simulink model "CRH2forBenchmark"  (R2014a)
settings: Solver=ode3  StartTime=0.0  StopTime=1  FixedStep=1e-5  RelTol=1e-3
PostLoadFcn:
  | , if any(exist('dsrtsu_mdlpostloadfcn', 'file') == [2, 3, 6]), try dsrtsu_mdlpostloadfcn('Execute', bdroot); catch fprintf('Error in PostLoadFcn (dsrtsu_mdlpostloadfcn) for model "%s":\n %s\n', bdroot, lasterr); end, end,
values from neighbouring files (symbols this model uses):
  Cd = 0.016    [CRH2forBenchmark.mat]
  Lm = 0.032848    [CRH2forBenchmark.mat]
  Ln = 0.002    [CRH2forBenchmark.mat]
  Lr = 0.034142    [CRH2forBenchmark.mat]
  Ls = 0.0342654    [CRH2forBenchmark.mat]
  np = 2    [CRH2forBenchmark.mat]
  Rd = 6000    [CRH2forBenchmark.mat]
  Rn = 0.2    [CRH2forBenchmark.mat]
  Rr = 0.146    [CRH2forBenchmark.mat]
  Rs = 0.144    [CRH2forBenchmark.mat]
  ts = 1e-05    [CRH2forBenchmark.mat]
undefined symbols (not defined in the file): J, KIM, KIT, KPM, KPT, phir, Ts, Vge
libraries: simulink x10
(part 1 of 3)
settings Model: DSRTSU_INTERNAL_RTI_VER=450  DSRTSU_INTERNAL_RTI_TYPE=rti1007  DSRTSU_INTERNAL_RTIFPGA=40  BufferReuse=off  Creator=超  LastModifiedBy=卍
settings SolverCC: AlgebraicLoopSolver=LineSearch
settings DataIOCC: SignalLoggingSaveFormat=ModelDataLogs
settings OptimizationCC: BlockReduction=off  OptimizeBlockIOStorage=off  BufferReuse=off  GlobalBufferReuse=off  ExpressionFolding=off  LocalBlockOutputs=off
settings DebuggingCC: MultiTaskDSMMsg=warning  MultiTaskCondExecSysMsg=none
settings HardwareCC: ProdIntDivRoundTo=Zero  ProdEndianess=BigEndian  ProdHWDeviceType=Generic->Custom  TargetIntDivRoundTo=Zero  TargetEndianess=BigEndian  TargetHWDeviceType=Generic->Custom
settings RTWCC: SystemTargetFile=rti1007.tlc  MakeCommand=make_rti  TemplateMakefile=rti1007.tmf  Description=dSPACE DS1007 Hardware Platform  ProcessScript=rti1007_make_rtw_hook  IncludeERTFirstTime=on
settings STFCustomTargetCC: ParMdlRefBuildCompliant=on  ConcurrentExecutionCompliant=off  MatFileLogging=on  SystemTargetFile=rti1007.tlc
settings GRTTargetCC: CompOptLevelCompliant=off  ConcurrentExecutionCompliant=off  CombineOutputUpdateFcns=off  CPPClassGenCompliant=off  GRTInterface=on  ExtModeMexFile=noextcomm

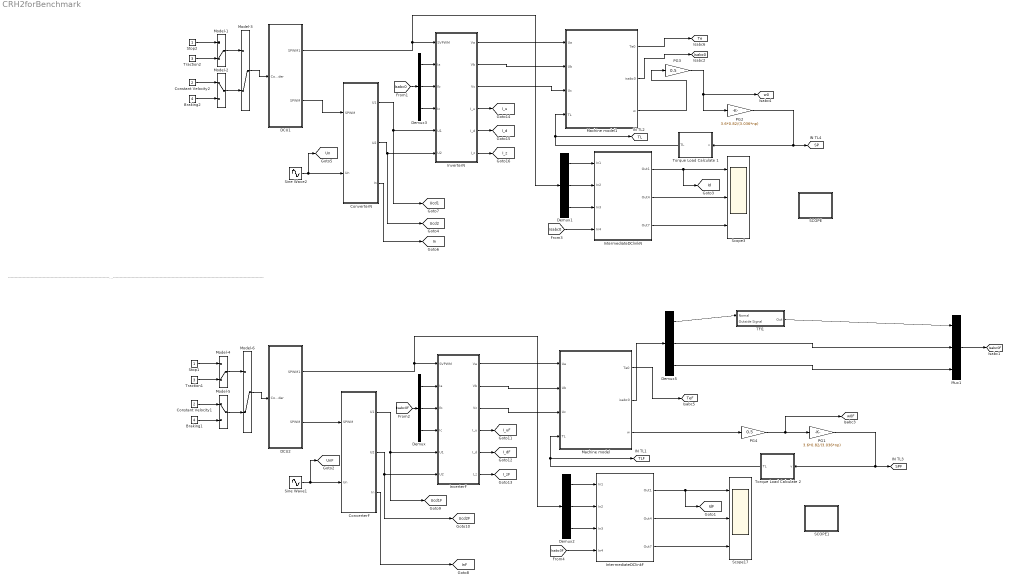
== system CRH2forBenchmark ==
  note: ------------------------------------------------------------------------------------------------------------------------------------------------------------------------------------------------------------------------------------------------------------------------------------------------------------------------------------------------------------------------------------------------------------------------------------------------------------------------------------------------------------------------------------------------------------------------------------------------------------------------------------------------------------------------------------------------------------------------------------------------------------------------------------------------------------------------------------------------------------------
  " Constant Velocity1" : Constant  Value=2
  " Constant Velocity2" : Constant  Value=2
  Braking1 : Constant  Value=4
  Braking2 : Constant  Value=4
  ConverterF : Subsystem
  ConverterN : Subsystem
  DCU1 : Subsystem  mask{sfcnParam1=KIM, sfcnParam2=KIT, sfcnParam3=KPM, sfcnParam4=KPT, sfcnParam5=Ts, sfcnParam6=Vge, sfcnParam7=np, sfcnParam8=phir}
      mask prompts: sfcnParam1 "KIM:"; sfcnParam2 "KIT:"; sfcnParam3 "KPM:"; sfcnParam4 "KPT:"; sfcnParam5 "Ts:"; sfcnParam6 "Vge:"; sfcnParam7 "np:"; sfcnParam8 "phir:"
      mask help: Simulink:masks:GenSFuncDesc_MD
      mask Help: eval('feval(''rtwprivate'',''rtwhelpview'',''rtw_sfcn_block'')');
      mask Display: fprintf('Traction Control\nUnit(TCU)')
  DCU2 : Subsystem  mask{sfcnParam1=KIM, sfcnParam2=KIT, sfcnParam3=KPM, sfcnParam4=KPT, sfcnParam5=Ts, sfcnParam6=Vge, sfcnParam7=np, sfcnParam8=phir}
      mask prompts: sfcnParam1 "KIM:"; sfcnParam2 "KIT:"; sfcnParam3 "KPM:"; sfcnParam4 "KPT:"; sfcnParam5 "Ts:"; sfcnParam6 "Vge:"; sfcnParam7 "np:"; sfcnParam8 "phir:"
      mask help: Simulink:masks:GenSFuncDesc_MD
      mask Help: eval('feval(''rtwprivate'',''rtwhelpview'',''rtw_sfcn_block'')');
      mask Display: fprintf('Traction Control\nUnit(TCU)')
  Demux{,1..3,5} (5 alike) : Demux  Outputs=3
  IntermediateDClinkF : Subsystem
      mask help: Simulink:masks:GenSFuncDesc_MD
      mask Help: eval('feval(''rtwprivate'',''rtwhelpview'',''rtw_sfcn_block'')');
  IntermediateDClinkN : Subsystem
      mask help: Simulink:masks:GenSFuncDesc_MD
      mask Help: eval('feval(''rtwprivate'',''rtwhelpview'',''rtw_sfcn_block'')');
  InverterF : Subsystem
  InverterN : Subsystem
  Machine model : Subsystem
  Machine model1 : Subsystem
  Model-{1,3..4,6} (4 alike) : ManualSwitch  CurrentSetting=0
  Model-2 : ManualSwitch
  Model-5 : ManualSwitch
  Mux1 : Mux  Inputs=3
  PG1 : Gain  Gain=3.6*0.82/(3.036*np)
  PG2 : Gain  Gain=3.6*0.82/(3.036*np)
  PG3 : Gain  Gain=0.5
  PG4 : Gain  Gain=0.5
  SCOPE : Subsystem
  SCOPE1 : Subsystem
  Scope17 : Scope  NumInputPorts=3
      settings: TickLabels=on  TimeRange=5  YMin=0~-110~-130  YMax=130~110~0  SaveName=AF  SampleInput=on  SampleTime=ts
  Scope3 : Scope  NumInputPorts=3
      settings: TickLabels=on  TimeRange=5  YMin=0~-110~-130  YMax=130~110~0  SaveName=A  SampleInput=on  SampleTime=ts
  Sine Wave1 : Sin  Amplitude=2121  Frequency=50*pi*2  SampleTime=ts
  Sine Wave2 : Sin  Amplitude=2121  Frequency=50*pi*2  SampleTime=ts
  Stop1 : Constant
  Stop2 : Constant
  TFI1 : Subsystem  mask(TFI){FaultType=SET anolog mode fault, FaultInjectionTime=1, Apq=[25 -500 -1000], TH=3.5, InvertBit=1, Register_Ts=1e-5, NoiseSelec=on, NoiseFault=[0.001 1e-5 23341], Comp_ConV=[23341], AddMux=Add}
      mask prompts: FaultType "Fault Type"; FaultInjectionTime "Fault Injection Time"; Apq "A,p,q"; InvertBit "Invert Bit"; NoiseSelec "Noise Disturbance"; NoiseFault "Noise Disturbance(Noise power,Sample time,Seed)"; Comp_ConV "Compare Constant Value"; AddMux "Add or Mux(outside signal)"
      mask help:
      | TCU Fault Injector (TFI)
      | 1.Fault Injection Time:Set the parameter of Fault-Inject Time;
      | 2.A,p,q:(Amplitude parameter, time parameter, time parameter)Setting analog model fault injection(Double exponential model ) signal by 3 parameter abvove
      | 3.TH: Threshold, Setting digital modle fault injecion
      | 4.Select Bit:Select number of data bits
      | 5.Invert Bit:Select the flip bit in register
      mask TypeOptions FaultType: Normal | SET anolog mode fault | SET digital mode fault | SRT register mode fault | Outside Signal
      mask TypeOptions InvertBit: 1 | 2 | 3 | 4 | 5 | 6 | 7 | 8 | 9 | 10 | 11 | 12 | 13 | 14 | 15 | 16
      mask TypeOptions AddMux: Add | Mux | Replace
      mask Display: fprintf('TCU Fault Injection')
  Torque Load Calculate 1 : Subsystem
  Torque Load Calculate 2 : Subsystem
  Traction1 : Constant  Value=3
  Traction2 : Constant  Value=3
  tag scope: I_d=global, I_dF=global, I_u=global, I_uF=global, I_z=global, I_zF=global, Id=global, IdF=global, In=global, InF=global, Isabc0=global, Isabc0F=global, SP=global, SPF=global, TL=global, TLF=global, Te=global, TeF=global, Ucd1=global, Ucd1F=global, Ucd2=global, Ucd2F=global, Un=global, UnF=global, w0=global, w0F=global
  wires:
  Stop1/1 -> Model-4/1
  Model-4/1 -> Model-6/1
  Model-5/1 -> Model-6/2
  Traction1/1 -> Model-4/2
  " Constant Velocity1"/1 -> Model-5/1
  Braking1/1 -> Model-5/2
  Model-6/1 -> DCU2/1(Commander)
  ConverterF/2(U2) -> [Ucd2F], InverterF/6(U2)
  ConverterF/1(U1) -> [Ucd1F], InverterF/5(U1)
  DCU2/2(SPWM) -> ConverterF/1(SPWM)
  DCU2/1(SPWM1) -> InverterF/1(SVPWM), Demux2/1
  Demux2/1 -> IntermediateDClinkF/1(In1)
  Demux2/2 -> IntermediateDClinkF/2(In2)
  Demux2/3 -> IntermediateDClinkF/3(In3)
  IntermediateDClinkF/2(Out4) -> Scope17/2
  IntermediateDClinkF/3(Out7) -> Scope17/3
  [Isabc0F] -> IntermediateDClinkF/4(In4)
  Sine Wave1/1 -> [UnF], ConverterF/2(Un)
  Torque Load Calculate 2/1(TL) -> [TLF], Machine model/4(TL)
  InverterF/1(Va) -> Machine model/1(Ua)
  InverterF/2(Vb) -> Machine model/2(Ub)
  InverterF/3(Vc) -> Machine model/3(Uc)
  PG4/1 -> PG1/1, [w0F]
  IntermediateDClinkF/1(Out1) -> [IdF], Scope17/1
  PG1/1 -> Torque Load Calculate 2/1(v), [SPF]
  Stop2/1 -> Model-1/1
  Model-1/1 -> Model-3/1
  Model-2/1 -> Model-3/2
  Traction2/1 -> Model-1/2
  " Constant Velocity2"/1 -> Model-2/1
  Braking2/1 -> Model-2/2
  Model-3/1 -> DCU1/1(Commander)
  ConverterN/2(U2) -> InverterN/6(U2), [Ucd2]
  ConverterN/1(U1) -> InverterN/5(U1), [Ucd1]
  DCU1/2(SPWM) -> ConverterN/1(SPWM)
  DCU1/1(SPWM1) -> InverterN/1(SVPWM), Demux1/1
  Demux1/1 -> IntermediateDClinkN/1(In1)
  Demux1/2 -> IntermediateDClinkN/2(In2)
  Demux1/3 -> IntermediateDClinkN/3(In3)
  IntermediateDClinkN/2(Out4) -> Scope3/2
  IntermediateDClinkN/3(Out7) -> Scope3/3
  [Isabc0] -> IntermediateDClinkN/4(In4)
  Sine Wave2/1 -> [Un], ConverterN/2(Un)
  ConverterN/3(In) -> [In]
  Torque Load Calculate 1/1(TL) -> Machine model1/4(TL), [TL]
  Machine model1/3(w) -> PG3/1
  InverterN/1(Va) -> Machine model1/1(Ua)
  InverterN/2(Vb) -> Machine model1/2(Ub)
  InverterN/3(Vc) -> Machine model1/3(Uc)
  PG3/1 -> PG2/1, [w0]
  IntermediateDClinkN/1(Out1) -> [Id], Scope3/1
  PG2/1 -> [SP], Torque Load Calculate 1/1(v)
  Machine model/2(isabc0) -> Demux5/1
  Mux1/1 -> [Isabc0F]
  Machine model1/2(isabc0) -> [Isabc0]
  Machine model/1(Te0) -> [TeF]
  Machine model1/1(Te0) -> [Te]
  Machine model/3(w) -> PG4/1
  Demux5/2 -> Mux1/2
  Demux5/3 -> Mux1/3
  InverterF/4(I_u) -> [I_uF]
  InverterF/5(I_d) -> [I_dF]
  InverterF/6(I_z) -> [I_zF]
  ConverterF/3(In) -> [InF]
  Demux/1 -> InverterF/2(Ia)
  Demux/2 -> InverterF/3(Ib)
  Demux/3 -> InverterF/4(Ic)
  [Isabc0F] -> Demux/1
  Demux3/1 -> InverterN/2(Ia)
  Demux3/2 -> InverterN/3(Ib)
  Demux3/3 -> InverterN/4(Ic)
  [Isabc0] -> Demux3/1
  InverterN/4(I_u) -> [I_u]
  InverterN/5(I_d) -> [I_d]
  InverterN/6(I_z) -> [I_z]
  Demux5/1 -> TFI1/1(Nomal)
  TFI1/1(Out) -> Mux1/1

== system CRH2forBenchmark/ConverterF ==
  SPWM : Inport
  Un : Inport  Port=2
  ConvDCLinkF : Subsystem
  Demux6 : Demux  Outputs=8
  Rectifier : Subsystem
  U1 : Outport
  U2 : Outport  Port=2
  In : Outport  Port=3
  tag scope: IABF=global, U1F=global, U2F=global, UNF=global
  wires:
  Demux6/3 -> Rectifier/3(Ta3)
  Demux6/4 -> Rectifier/4(Ta4)
  Demux6/1 -> Rectifier/1(Ta1)
  Demux6/6 -> Rectifier/6(Tb2)
  Demux6/5 -> Rectifier/5(Tb1)
  Rectifier/4(Id) -> ConvDCLinkF/2(ID)
  Rectifier/2(Iu) -> ConvDCLinkF/1(IU)
  Rectifier/1(In*) -> Rectifier/9(In), In/1, [IABF]
  SPWM/1 -> Demux6/1
  Demux6/8 -> Rectifier/8(Tb4)
  Demux6/7 -> Rectifier/7(Tb3)
  Un/1 -> [UNF], Rectifier/12(Un)
  ConvDCLinkF/1(U1*) -> [U1F], U1/1, Rectifier/10(U1), ConvDCLinkF/3(U1)
  ConvDCLinkF/2(U2*) -> [U2F], U2/1, Rectifier/11(U2), ConvDCLinkF/4(U2)
  Demux6/2 -> Rectifier/2(Ta2)

== system CRH2forBenchmark/ConverterN ==
  SPWM : Inport
  Un : Inport  Port=2
  Demux : Demux  Outputs=8
  Rectifier : Subsystem
  Subsystem : Subsystem
  U1 : Outport
  U2 : Outport  Port=2
  In : Outport  Port=3
  tag scope: IAB=global, U1=global, U2=global, UN=global
  wires:
  Subsystem/2(U2*) -> Subsystem/4(U2), Rectifier/11(U2), U2/1, [U2]
  Subsystem/1(U1*) -> Subsystem/3(U1), Rectifier/10(U1), U1/1, [U1]
  Un/1 -> Rectifier/12(Un), [UN]
  Demux/7 -> Rectifier/7(Tb3)
  Demux/8 -> Rectifier/8(Tb4)
  SPWM/1 -> Demux/1
  Rectifier/1(In*) -> [IAB], In/1, Rectifier/9(In)
  Rectifier/2(Iu) -> Subsystem/1(IU)
  Rectifier/4(Id) -> Subsystem/2(ID)
  Demux/5 -> Rectifier/5(Tb1)
  Demux/6 -> Rectifier/6(Tb2)
  Demux/1 -> Rectifier/1(Ta1)
  Demux/4 -> Rectifier/4(Ta4)
  Demux/2 -> Rectifier/2(Ta2)
  Demux/3 -> Rectifier/3(Ta3)

== system CRH2forBenchmark/DCU1 ==
  Commander : Inport
  DCU1_sfcn : S-Function  FunctionName=DCU1_sf  Parameters=sfcnParam1, sfcnParam2, sfcnParam3, sfcnParam4, sfcnParam5, sfcnParam6, sfcnParam7, sfcnParam8  SFunctionModules=""  EnableBusSupport=off  mask{rtw_sf_name=DCU1_sf, showVar=off, sfcnParam1=sfcnParam1, sfcnParam2=sfcnParam2, sfcnParam3=sfcnParam3, sfcnParam4=sfcnParam4, sfcnParam5=sfcnParam5, sfcnParam6=sfcnParam6, sfcnParam7=sfcnParam7, sfcnParam8=sfcnParam8}
      mask prompts: rtw_sf_name "Simulink:masks:GenSFuncName_MP"; showVar "Simulink:masks:GenSFuncShowModuleList_MP"; sfcnParam1 "KIM:"; sfcnParam2 "KIT:"; sfcnParam3 "KPM:"; sfcnParam4 "KPT:"; sfcnParam5 "Ts:"; sfcnParam6 "Vge:"; sfcnParam7 "np:"; sfcnParam8 "phir:"
      mask help: Simulink:masks:GenSFuncDesc_MD
      mask init:
      | displist = '';
      | if ~strcmp(get_param(gcb, 'FunctionName'), rtw_sf_name);
      |   set_param(gcb, 'FunctionName', rtw_sf_name);
      | end
      | % Check if we are generating code
      | rtw_mode = false;
      | if strcmpi(get_param(bdroot(gcb),'SimulationStatus'),'Initializing')
      | 	rtw_mode = strcmpi(get_param(bdroot(gcb),'BuildingRTWCode'),'on') && ...
      | 		~strcmpi(get_param(bdroot(gcb),'TargetStyle'),'SimulationTarget');
      | end
      | if showVar || rtw_mode
      | 	if exist('rtwsfunc') == 2 | exist('rtwsfunc') == 6
      | 		tmplist = rtwsfunc(rtw_sf_name,gcb);
      | 		tmplist = DAStudio.message('Simulink:masks:GenSFuncListOfModules_IC', tmplist);
      | 	elseif showVar
      | 		tmplist1 = DAStudio.message('Simulink:masks:GenSFuncListOfModules_IC', '');
      |         tmplist2 = DAStudio.message('Simulink:masks:GenSFuncNotLicensed_IC');
      |         tmplist = [tmplist1 tmplist2];
      |  	end
      | end
      | if showVar
      |   displist = tmplist;
      | end
      settings: CopyFcn=|
      | if ~strcmp(get_param(gcb,'Linkstatus'),'none') && ...
      | ~strcmp(get_param(gcb,'Linkstatus'),'implicit')
      |   set_param(gcb,'LinkStatus','none');
      | end
      mask Help: eval('feval(''rtwprivate'',''rtwhelpview'',''rtw_sfcn_block'')');
      mask Display:
      | port_label('input',1,'Commander');
      | port_label('input',2,'Inport1');
      | port_label('input',3,'Inport2');
      | port_label('input',4,'Inport3');
      | port_label('input',5,'Inport4');
      | port_label('input',6,'Inport5');
      | port_label('input',7,'Inport6');
      | port_label('input',8,'Inport7');
      | port_label('input',9,'Inport8');
      | port_label('output',1,'SPWM1');
      | port_label('output',2,'SPWM');
  __InputSSForSFun__ : Subsystem
  __OutputSSForSFun__ : Subsystem
  SPWM1 : Outport
  SPWM : Outport  Port=2
  wires:
  __OutputSSForSFun__/2(SPWM) -> SPWM/1
  __OutputSSForSFun__/1(SPWM1) -> SPWM1/1
  DCU1_sfcn/2 -> __OutputSSForSFun__/2(__UniqueInportName__2__)
  DCU1_sfcn/1 -> __OutputSSForSFun__/1(__UniqueInportName__1__)
  __InputSSForSFun__/9(__UniqueOutportName__9__) -> DCU1_sfcn/9
  __InputSSForSFun__/8(__UniqueOutportName__8__) -> DCU1_sfcn/8
  __InputSSForSFun__/7(__UniqueOutportName__7__) -> DCU1_sfcn/7
  __InputSSForSFun__/6(__UniqueOutportName__6__) -> DCU1_sfcn/6
  __InputSSForSFun__/5(__UniqueOutportName__5__) -> DCU1_sfcn/5
  __InputSSForSFun__/4(__UniqueOutportName__4__) -> DCU1_sfcn/4
  __InputSSForSFun__/3(__UniqueOutportName__3__) -> DCU1_sfcn/3
  __InputSSForSFun__/2(__UniqueOutportName__2__) -> DCU1_sfcn/2
  __InputSSForSFun__/1(__UniqueOutportName__1__) -> DCU1_sfcn/1
  Commander/1 -> __InputSSForSFun__/1(Commander)

== system CRH2forBenchmark/DCU2 ==
  Commander : Inport
  DCU2_sfcn : S-Function  FunctionName=DCU2_sf  Parameters=sfcnParam1, sfcnParam2, sfcnParam3, sfcnParam4, sfcnParam5, sfcnParam6, sfcnParam7, sfcnParam8  SFunctionModules=""  EnableBusSupport=off  mask{rtw_sf_name=DCU2_sf, showVar=off, sfcnParam1=sfcnParam1, sfcnParam2=sfcnParam2, sfcnParam3=sfcnParam3, sfcnParam4=sfcnParam4, sfcnParam5=sfcnParam5, sfcnParam6=sfcnParam6, sfcnParam7=sfcnParam7, sfcnParam8=sfcnParam8}
      mask prompts: rtw_sf_name "Simulink:masks:GenSFuncName_MP"; showVar "Simulink:masks:GenSFuncShowModuleList_MP"; sfcnParam1 "KIM:"; sfcnParam2 "KIT:"; sfcnParam3 "KPM:"; sfcnParam4 "KPT:"; sfcnParam5 "Ts:"; sfcnParam6 "Vge:"; sfcnParam7 "np:"; sfcnParam8 "phir:"
      mask help: Simulink:masks:GenSFuncDesc_MD
      mask init: same as CRH2forBenchmark/DCU1/DCU1_sfcn
      settings: CopyFcn=|
      | if ~strcmp(get_param(gcb,'Linkstatus'),'none') && ...
      | ~strcmp(get_param(gcb,'Linkstatus'),'implicit')
      |   set_param(gcb,'LinkStatus','none');
      | end
      mask Help: eval('feval(''rtwprivate'',''rtwhelpview'',''rtw_sfcn_block'')');
      mask Display:
      | port_label('input',1,'Commander');
      | port_label('input',2,'Inport1');
      | port_label('input',3,'Inport2');
      | port_label('input',4,'Inport3');
      | port_label('input',5,'Inport4');
      | port_label('input',6,'Inport5');
      | port_label('input',7,'Inport6');
      | port_label('input',8,'Inport7');
      | port_label('input',9,'Inport8');
      | port_label('output',1,'SPWM1');
      | port_label('output',2,'SPWM');
  __InputSSForSFun__ : Subsystem
  __OutputSSForSFun__ : Subsystem
  SPWM1 : Outport
  SPWM : Outport  Port=2
  wires:
  Commander/1 -> __InputSSForSFun__/1(Commander)
  __InputSSForSFun__/1(__UniqueOutportName__1__) -> DCU2_sfcn/1
  __InputSSForSFun__/2(__UniqueOutportName__2__) -> DCU2_sfcn/2
  __InputSSForSFun__/3(__UniqueOutportName__3__) -> DCU2_sfcn/3
  __InputSSForSFun__/4(__UniqueOutportName__4__) -> DCU2_sfcn/4
  __InputSSForSFun__/5(__UniqueOutportName__5__) -> DCU2_sfcn/5
  __InputSSForSFun__/6(__UniqueOutportName__6__) -> DCU2_sfcn/6
  __InputSSForSFun__/7(__UniqueOutportName__7__) -> DCU2_sfcn/7
  __InputSSForSFun__/8(__UniqueOutportName__8__) -> DCU2_sfcn/8
  __InputSSForSFun__/9(__UniqueOutportName__9__) -> DCU2_sfcn/9
  DCU2_sfcn/1 -> __OutputSSForSFun__/1(__UniqueInportName__1__)
  DCU2_sfcn/2 -> __OutputSSForSFun__/2(__UniqueInportName__2__)
  __OutputSSForSFun__/1(SPWM1) -> SPWM1/1
  __OutputSSForSFun__/2(SPWM) -> SPWM/1

== system CRH2forBenchmark/IntermediateDClinkF ==
  In1 : Inport
  In2 : Inport  Port=2
  In3 : Inport  Port=3
  In4 : Inport  Port=4
  IntermediateDClinkF_sfcn : S-Function  FunctionName=IntermediateDClinkF_sf  SFunctionModules=""  EnableBusSupport=off  mask{rtw_sf_name=IntermediateDClinkF_sf, showVar=off}
      mask prompts: rtw_sf_name "Simulink:masks:GenSFuncName_MP"; showVar "Simulink:masks:GenSFuncShowModuleList_MP"
      mask help: Simulink:masks:GenSFuncDesc_MD
      mask init: same as CRH2forBenchmark/DCU1/DCU1_sfcn
      settings: CopyFcn=|
      | if ~strcmp(get_param(gcb,'Linkstatus'),'none') && ...
      | ~strcmp(get_param(gcb,'Linkstatus'),'implicit')
      |   set_param(gcb,'LinkStatus','none');
      | end
      mask Help: eval('feval(''rtwprivate'',''rtwhelpview'',''rtw_sfcn_block'')');
      mask Display:
      | port_label('input',1,'In1');
      | port_label('input',2,'In2');
      | port_label('input',3,'In3');
      | port_label('input',4,'In4');
      | port_label('output',1,'Out1');
      | port_label('output',2,'Out4');
      | port_label('output',3,'Out7');
  __InputSSForSFun__ : Subsystem
  __OutputSSForSFun__ : Subsystem
  Out1 : Outport
  Out4 : Outport  Port=2
  Out7 : Outport  Port=3
  wires:
  In1/1 -> __InputSSForSFun__/1(In1)
  In2/1 -> __InputSSForSFun__/2(In2)
  In3/1 -> __InputSSForSFun__/3(In3)
  In4/1 -> __InputSSForSFun__/4(In4)
  __InputSSForSFun__/1(__UniqueOutportName__1__) -> IntermediateDClinkF_sfcn/1
  __InputSSForSFun__/2(__UniqueOutportName__2__) -> IntermediateDClinkF_sfcn/2
  __InputSSForSFun__/3(__UniqueOutportName__3__) -> IntermediateDClinkF_sfcn/3
  __InputSSForSFun__/4(__UniqueOutportName__4__) -> IntermediateDClinkF_sfcn/4
  IntermediateDClinkF_sfcn/1 -> __OutputSSForSFun__/1(__UniqueInportName__1__)
  IntermediateDClinkF_sfcn/2 -> __OutputSSForSFun__/2(__UniqueInportName__2__)
  IntermediateDClinkF_sfcn/3 -> __OutputSSForSFun__/3(__UniqueInportName__3__)
  __OutputSSForSFun__/1(Out1) -> Out1/1
  __OutputSSForSFun__/2(Out4) -> Out4/1
  __OutputSSForSFun__/3(Out7) -> Out7/1

== system CRH2forBenchmark/IntermediateDClinkN ==
  In1 : Inport
  In2 : Inport  Port=2
  In3 : Inport  Port=3
  In4 : Inport  Port=4
  IntermediateDClinkN_sfcn : S-Function  FunctionName=IntermediateDClinkN_sf  SFunctionModules=""  EnableBusSupport=off  mask{rtw_sf_name=IntermediateDClinkN_sf, showVar=off}
      mask prompts: rtw_sf_name "Simulink:masks:GenSFuncName_MP"; showVar "Simulink:masks:GenSFuncShowModuleList_MP"
      mask help: Simulink:masks:GenSFuncDesc_MD
      mask init: same as CRH2forBenchmark/DCU1/DCU1_sfcn
      settings: CopyFcn=|
      | if ~strcmp(get_param(gcb,'Linkstatus'),'none') && ...
      | ~strcmp(get_param(gcb,'Linkstatus'),'implicit')
      |   set_param(gcb,'LinkStatus','none');
      | end
      mask Help: eval('feval(''rtwprivate'',''rtwhelpview'',''rtw_sfcn_block'')');
      mask Display:
      | port_label('input',1,'In1');
      | port_label('input',2,'In2');
      | port_label('input',3,'In3');
      | port_label('input',4,'In4');
      | port_label('output',1,'Out1');
      | port_label('output',2,'Out4');
      | port_label('output',3,'Out7');
  __InputSSForSFun__ : Subsystem
  __OutputSSForSFun__ : Subsystem
  Out1 : Outport
  Out4 : Outport  Port=2
  Out7 : Outport  Port=3
  wires:
  In1/1 -> __InputSSForSFun__/1(In1)
  In2/1 -> __InputSSForSFun__/2(In2)
  In3/1 -> __InputSSForSFun__/3(In3)
  In4/1 -> __InputSSForSFun__/4(In4)
  __InputSSForSFun__/1(__UniqueOutportName__1__) -> IntermediateDClinkN_sfcn/1
  __InputSSForSFun__/2(__UniqueOutportName__2__) -> IntermediateDClinkN_sfcn/2
  __InputSSForSFun__/3(__UniqueOutportName__3__) -> IntermediateDClinkN_sfcn/3
  __InputSSForSFun__/4(__UniqueOutportName__4__) -> IntermediateDClinkN_sfcn/4
  IntermediateDClinkN_sfcn/1 -> __OutputSSForSFun__/1(__UniqueInportName__1__)
  IntermediateDClinkN_sfcn/2 -> __OutputSSForSFun__/2(__UniqueInportName__2__)
  IntermediateDClinkN_sfcn/3 -> __OutputSSForSFun__/3(__UniqueInportName__3__)
  __OutputSSForSFun__/1(Out1) -> Out1/1
  __OutputSSForSFun__/2(Out4) -> Out4/1
  __OutputSSForSFun__/3(Out7) -> Out7/1

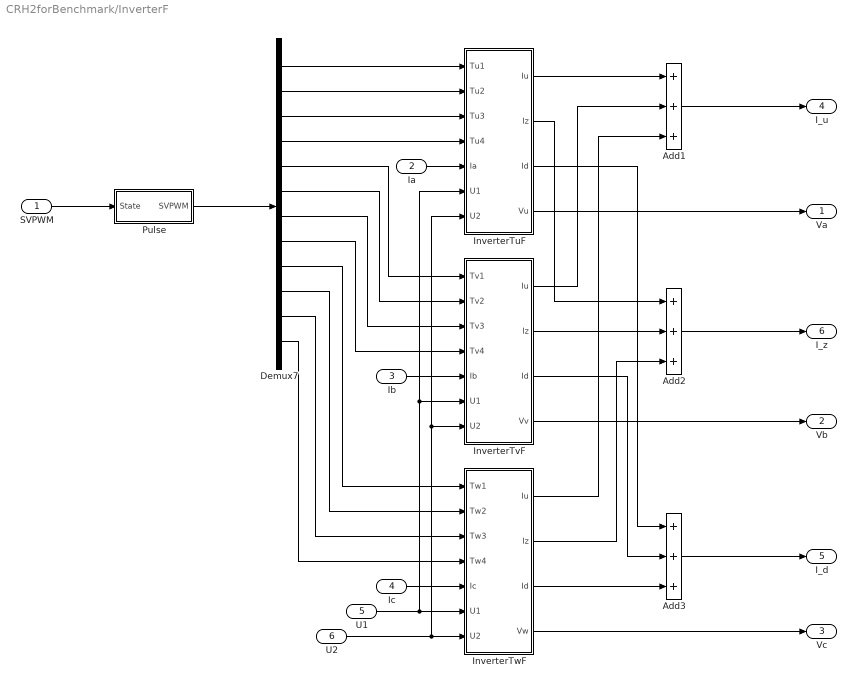
== system CRH2forBenchmark/InverterF ==
  SVPWM : Inport
  Ia : Inport  Port=2
  Ib : Inport  Port=3
  Ic : Inport  Port=4
  U1 : Inport  Port=5
  U2 : Inport  Port=6
  Add1 : Sum  Inputs=+++  SampleTime=ts
  Add2 : Sum  Inputs=+++  SampleTime=ts
  Add3 : Sum  Inputs=+++  SampleTime=ts
  Demux7 : Demux  Outputs=12
  InverterTuF : Subsystem
      mask help: Simulink:masks:GenSFuncDesc_MD
      mask Help: eval('feval(''rtwprivate'',''rtwhelpview'',''rtw_sfcn_block'')');
  InverterTvF : Subsystem
      mask help: Simulink:masks:GenSFuncDesc_MD
      mask Help: eval('feval(''rtwprivate'',''rtwhelpview'',''rtw_sfcn_block'')');
  InverterTwF : Subsystem
      mask help: Simulink:masks:GenSFuncDesc_MD
      mask Help: eval('feval(''rtwprivate'',''rtwhelpview'',''rtw_sfcn_block'')');
  Pulse : Subsystem
  Va : Outport
  Vb : Outport  Port=2
  Vc : Outport  Port=3
  I_u : Outport  Port=4
  I_d : Outport  Port=5
  I_z : Outport  Port=6
  wires:
  Demux7/1 -> InverterTuF/1(Tu1)
  Demux7/2 -> InverterTuF/2(Tu2)
  Ia/1 -> InverterTuF/5(Ia)
  Add2/1 -> I_z/1
  Demux7/10 -> InverterTwF/2(Tw2)
  Ic/1 -> InverterTwF/5(Ic)
  Demux7/8 -> InverterTvF/4(Tv4)
  Demux7/9 -> InverterTwF/1(Tw1)
  InverterTwF/4(Vw) -> Vc/1
  U1/1 -> InverterTwF/6(U1), InverterTvF/6(U1), InverterTuF/6(U1)
  SVPWM/1 -> Pulse/1(State)
  Demux7/6 -> InverterTvF/2(Tv2)
  Demux7/11 -> InverterTwF/3(Tw3)
  Demux7/12 -> InverterTwF/4(Tw4)
  InverterTvF/4(Vv) -> Vb/1
  InverterTwF/3(Id) -> Add3/3
  Demux7/4 -> InverterTuF/4(Tu4)
  Add1/1 -> I_u/1
  Demux7/7 -> InverterTvF/3(Tv3)
  InverterTuF/3(Id) -> Add3/1
  Demux7/5 -> InverterTvF/1(Tv1)
  Demux7/3 -> InverterTuF/3(Tu3)
  Ib/1 -> InverterTvF/5(Ib)
  U2/1 -> InverterTwF/7(U2), InverterTvF/7(U2), InverterTuF/7(U2)
  InverterTuF/4(Vu) -> Va/1
  InverterTvF/3(Id) -> Add3/2
  Add3/1 -> I_d/1
  InverterTwF/1(Iu) -> Add1/3
  InverterTvF/2(Iz) -> Add2/2
  InverterTuF/1(Iu) -> Add1/1
  InverterTuF/2(Iz) -> Add2/1
  InverterTwF/2(Iz) -> Add2/3
  InverterTvF/1(Iu) -> Add1/2
  Pulse/1(SVPWM) -> Demux7/1

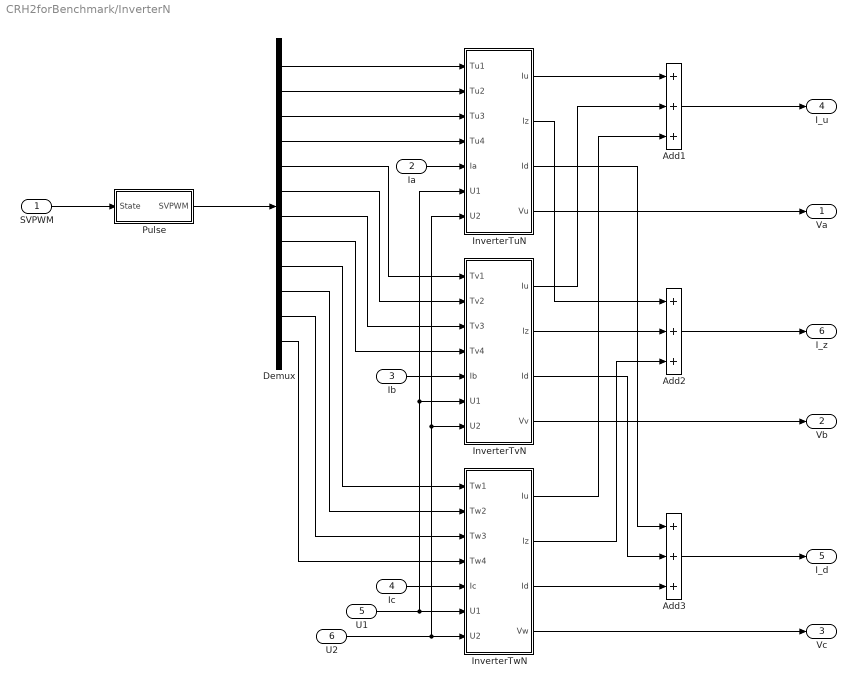
== system CRH2forBenchmark/InverterN ==
  SVPWM : Inport
  Ia : Inport  Port=2
  Ib : Inport  Port=3
  Ic : Inport  Port=4
  U1 : Inport  Port=5
  U2 : Inport  Port=6
  Add1 : Sum  Inputs=+++  SampleTime=ts
  Add2 : Sum  Inputs=+++  SampleTime=ts
  Add3 : Sum  Inputs=+++  SampleTime=ts
  Demux : Demux  Outputs=12
  InverterTuN : Subsystem
      mask help: Simulink:masks:GenSFuncDesc_MD
      mask Help: eval('feval(''rtwprivate'',''rtwhelpview'',''rtw_sfcn_block'')');
  InverterTvN : Subsystem
      mask help: Simulink:masks:GenSFuncDesc_MD
      mask Help: eval('feval(''rtwprivate'',''rtwhelpview'',''rtw_sfcn_block'')');
  InverterTwN : Subsystem
      mask help: Simulink:masks:GenSFuncDesc_MD
      mask Help: eval('feval(''rtwprivate'',''rtwhelpview'',''rtw_sfcn_block'')');
  Pulse : Subsystem
  Va : Outport
  Vb : Outport  Port=2
  Vc : Outport  Port=3
  I_u : Outport  Port=4
  I_d : Outport  Port=5
  I_z : Outport  Port=6
  wires:
  Pulse/1(SVPWM) -> Demux/1
  InverterTvN/1(Iu) -> Add1/2
  InverterTwN/2(Iz) -> Add2/3
  InverterTuN/2(Iz) -> Add2/1
  InverterTuN/1(Iu) -> Add1/1
  InverterTvN/2(Iz) -> Add2/2
  InverterTwN/1(Iu) -> Add1/3
  Add3/1 -> I_d/1
  InverterTvN/3(Id) -> Add3/2
  InverterTuN/4(Vu) -> Va/1
  U2/1 -> InverterTwN/7(U2), InverterTvN/7(U2), InverterTuN/7(U2)
  Ib/1 -> InverterTvN/5(Ib)
  Demux/3 -> InverterTuN/3(Tu3)
  Demux/5 -> InverterTvN/1(Tv1)
  InverterTuN/3(Id) -> Add3/1
  Demux/7 -> InverterTvN/3(Tv3)
  Add1/1 -> I_u/1
  Demux/4 -> InverterTuN/4(Tu4)
  InverterTwN/3(Id) -> Add3/3
  InverterTvN/4(Vv) -> Vb/1
  Demux/12 -> InverterTwN/4(Tw4)
  Demux/11 -> InverterTwN/3(Tw3)
  Demux/6 -> InverterTvN/2(Tv2)
  SVPWM/1 -> Pulse/1(State)
  U1/1 -> InverterTwN/6(U1), InverterTvN/6(U1), InverterTuN/6(U1)
  InverterTwN/4(Vw) -> Vc/1
  Demux/9 -> InverterTwN/1(Tw1)
  Demux/8 -> InverterTvN/4(Tv4)
  Ic/1 -> InverterTwN/5(Ic)
  Demux/10 -> InverterTwN/2(Tw2)
  Add2/1 -> I_z/1
  Ia/1 -> InverterTuN/5(Ia)
  Demux/2 -> InverterTuN/2(Tu2)
  Demux/1 -> InverterTuN/1(Tu1)

== system CRH2forBenchmark/Machine model ==
  Ua : Inport
  Ub : Inport  Port=2
  Uc : Inport  Port=3
  TL : Inport  Port=4
  Normal ModelF : Subsystem
  Step : Step  Time=1000  Before=1  After=0  SampleTime=0
  Switch : Switch  Criteria=u2 > Threshold
  Switch1 : Switch  Criteria=u2 > Threshold
  Switch2 : Switch  Criteria=u2 > Threshold
  Te0 : Outport
  isabc0 : Outport  Port=2
  w : Outport  Port=3
  wires:
  Normal ModelF/2(Isabc0) -> Switch1/1
  Normal ModelF/1(Te0) -> Switch/1
  Uc/1 -> Normal ModelF/3(Uc)
  Switch/1 -> Te0/1
  Switch1/1 -> isabc0/1
  Step/1 -> Switch2/2, Switch1/2, Switch/2
  Switch2/1 -> w/1
  Ub/1 -> Normal ModelF/2(Ub)
  TL/1 -> Normal ModelF/4(TL)
  Ua/1 -> Normal ModelF/1(Ua)
  Normal ModelF/3(w) -> Switch2/1

== system CRH2forBenchmark/Machine model1 ==
  Ua : Inport
  Ub : Inport  Port=2
  Uc : Inport  Port=3
  TL : Inport  Port=4
  Normal ModelN : Subsystem
  Step : Step  Time=1000  Before=1  After=0  SampleTime=0
  Switch : Switch  Criteria=u2 > Threshold
  Switch1 : Switch  Criteria=u2 > Threshold
  Switch2 : Switch  Criteria=u2 > Threshold
  Te0 : Outport
  isabc0 : Outport  Port=2
  w : Outport  Port=3
  wires:
  Normal ModelN/2(Isabc0) -> Switch1/1
  Normal ModelN/1(Te0) -> Switch/1
  Uc/1 -> Normal ModelN/3(Uc)
  Switch/1 -> Te0/1
  Switch1/1 -> isabc0/1
  Step/1 -> Switch2/2, Switch1/2, Switch/2
  Switch2/1 -> w/1
  Ub/1 -> Normal ModelN/2(Ub)
  TL/1 -> Normal ModelN/4(TL)
  Ua/1 -> Normal ModelN/1(Ua)
  Normal ModelN/3(w) -> Switch2/1

== system CRH2forBenchmark/SCOPE ==
  note: Ucd2
  note: Ucd1
  note: Isa
  note: Isb
  note: Isc
  Demux : Demux  Outputs=3
  Isa/Isb/Isc : Scope  NumInputPorts=3
      settings: ShowLegends=on  TimeRange=3  YMin=-220~-220~-220  YMax=220~220~220  SaveName=Ii  SampleTime=1e-5
  Sp/Rs/Te : Scope  NumInputPorts=3
      settings: TickLabels=on  TimeRange=5  YMin=0~-110~-130  YMax=130~110~0  SaveName=S  SampleInput=on  SampleTime=ts
  Ucd1/Ucd2 : Scope  NumInputPorts=2
      settings: ShowLegends=on  TimeRange=3  YMin=1285~1282.5  YMax=1315~1312.5  SaveName=Ucd  SampleTime=1e-5
  Un/In : Scope  NumInputPorts=2
      settings: TimeRange=3  YMin=-2500~-500  YMax=2500~500  SaveName=Un  SampleTime=1e-5
  wires:
  [Isabc0] -> Demux/1
  [Ucd1] -> Ucd1/Ucd2/1
  [Ucd2] -> Ucd1/Ucd2/2
  [UN] -> Un/In/1
  [In] -> Un/In/2
  Demux/2 -> Isa/Isb/Isc/2
  Demux/1 -> Isa/Isb/Isc/1
  Demux/3 -> Isa/Isb/Isc/3
  [Te] -> Sp/Rs/Te/3
  [w0] -> Sp/Rs/Te/2
  [SP] -> Sp/Rs/Te/1

== system CRH2forBenchmark/SCOPE1 ==
  note: Isa
  note: Isc
  note: Ucd2
  note: Ucd1
  note: Isb
  Demux : Demux  Outputs=3
  IsaF/IsbF/IscF : Scope  NumInputPorts=3
      settings: ShowLegends=on  TimeRange=3  YMin=-220~-220~-220  YMax=220~220~220  SaveName=IiF  SampleTime=1e-5
  SpF/RsF/TeF : Scope  NumInputPorts=3
      settings: TickLabels=on  TimeRange=5  YMin=0~-110~-130  YMax=130~110~0  SaveName=SF  SampleInput=on  SampleTime=ts
  UcdF1/UcdF2 : Scope  NumInputPorts=2
      settings: ShowLegends=on  TimeRange=1  YMin=1277.5~1277.5  YMax=1317.5~1315  SaveName=UcdF  SampleTime=1e-5
  UnF/InF : Scope  NumInputPorts=2
      settings: TimeRange=3  YMin=-2250~-400  YMax=2250~450  SaveName=UnF  SampleTime=1e-5
  wires:
  [Isabc0F] -> Demux/1
  [UNF] -> UnF/InF/1
  [InF] -> UnF/InF/2
  Demux/2 -> IsaF/IsbF/IscF/2
  Demux/1 -> IsaF/IsbF/IscF/1
  Demux/3 -> IsaF/IsbF/IscF/3
  [TeF] -> SpF/RsF/TeF/3
  [w0F] -> SpF/RsF/TeF/2
  [SPF] -> SpF/RsF/TeF/1
  [Ucd1F] -> UcdF1/UcdF2/1
  [Ucd2F] -> UcdF1/UcdF2/2

== system CRH2forBenchmark/TFI1 ==
  Nomal : Inport
  Outside Signal : Inport  Port=2
  TFI1Sub : Subsystem
  Out : Outport
  wires:
  TFI1Sub/1(Out) -> Out/1
  Outside Signal/1 -> TFI1Sub/2(Outside Signal)
  Nomal/1 -> TFI1Sub/1(Nomal)

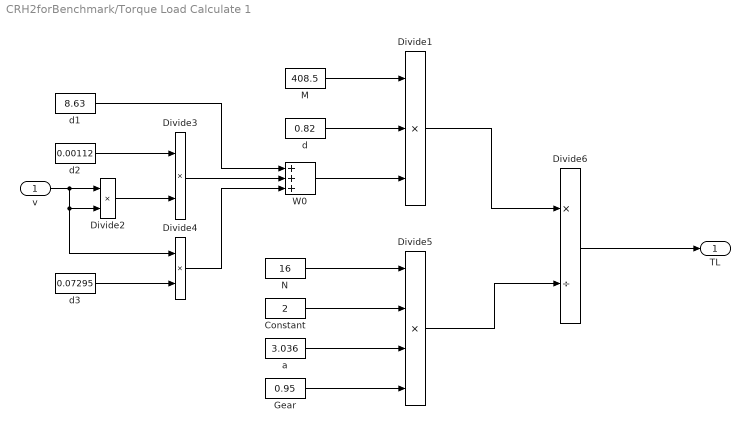
== system CRH2forBenchmark/Torque Load Calculate 1 ==
  v : Inport
  Constant : Constant  Value=2
  Divide1 : Product  Inputs=***
  Divide2 : Product  Inputs=**
  Divide3 : Product  Inputs=**
  Divide4 : Product  Inputs=**
  Divide5 : Product  Inputs=****
  Divide6 : Product  Inputs=*/
  Gear : Constant  Value=0.95
  M : Constant  Value=408.5
  N : Constant  Value=16
  W0 : Sum  Inputs=+++
  a : Constant  Value=3.036
  d : Constant  Value=0.82
  d1 : Constant  Value=8.63
  d2 : Constant  Value=0.00112
  d3 : Constant  Value=0.07295
  TL : Outport
  wires:
  Divide6/1 -> TL/1
  Divide5/1 -> Divide6/2
  Divide1/1 -> Divide6/1
  Gear/1 -> Divide5/4
  a/1 -> Divide5/3
  Constant/1 -> Divide5/2
  N/1 -> Divide5/1
  W0/1 -> Divide1/3
  Divide4/1 -> W0/3
  Divide3/1 -> W0/2
  d1/1 -> W0/1
  d3/1 -> Divide4/2
  d2/1 -> Divide3/1
  Divide2/1 -> Divide3/2
  v/1 -> Divide2/1, Divide2/2, Divide4/1
  d/1 -> Divide1/2
  M/1 -> Divide1/1

== system CRH2forBenchmark/Torque Load Calculate 2 ==
  v : Inport
  Constant : Constant  Value=2
  Divide1 : Product  Inputs=***
  Divide2 : Product  Inputs=**
  Divide3 : Product  Inputs=**
  Divide4 : Product  Inputs=**
  Divide5 : Product  Inputs=****
  Divide6 : Product  Inputs=*/
  Gear : Constant  Value=0.95
  M : Constant  Value=408.5
  N : Constant  Value=16
  W0 : Sum  Inputs=+++
  a : Constant  Value=3.036
  d : Constant  Value=0.82
  d1 : Constant  Value=8.63
  d2 : Constant  Value=0.00112
  d3 : Constant  Value=0.07295
  TL : Outport
  wires:
  Divide6/1 -> TL/1
  Divide5/1 -> Divide6/2
  Divide1/1 -> Divide6/1
  Gear/1 -> Divide5/4
  a/1 -> Divide5/3
  Constant/1 -> Divide5/2
  N/1 -> Divide5/1
  W0/1 -> Divide1/3
  Divide4/1 -> W0/3
  Divide3/1 -> W0/2
  d1/1 -> W0/1
  d3/1 -> Divide4/2
  d2/1 -> Divide3/1
  Divide2/1 -> Divide3/2
  v/1 -> Divide2/1, Divide2/2, Divide4/1
  d/1 -> Divide1/2
  M/1 -> Divide1/1

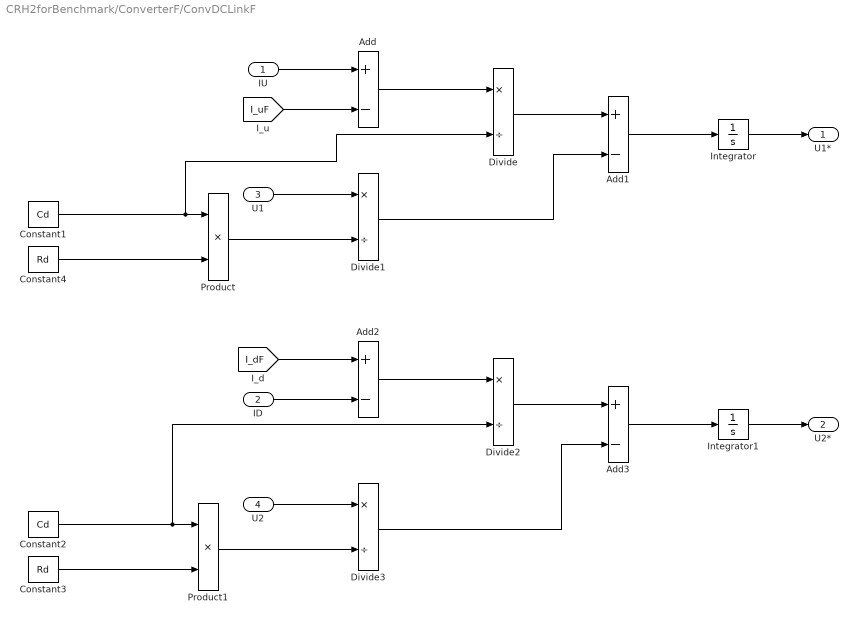
== system CRH2forBenchmark/ConverterF/ConvDCLinkF ==
  IU : Inport
  ID : Inport  Port=2
  U1 : Inport  Port=3
  U2 : Inport  Port=4
  Add{,1..3} (4 alike) : Sum  Inputs=+-  SampleTime=ts
  Constant1 : Constant  Value=Cd
  Constant2 : Constant  Value=Cd
  Constant3 : Constant  Value=Rd
  Constant4 : Constant  Value=Rd
  Divide{,1..3} (4 alike) : Product  Inputs=*/
  Integrator : Integrator
  Integrator1 : Integrator
  Product : Product  SampleTime=ts
  Product1 : Product  SampleTime=ts
  U1* : Outport
  U2* : Outport  Port=2
  wires:
  Add3/1 -> Integrator1/1
  Divide3/1 -> Add3/2
  Divide2/1 -> Add3/1
  U2/1 -> Divide3/1
  Product1/1 -> Divide3/2
  Add2/1 -> Divide2/1
  Constant2/1 -> Divide2/2, Product1/1
  [I_dF] -> Add2/1
  ID/1 -> Add2/2
  Add1/1 -> Integrator/1
  Divide1/1 -> Add1/2
  Divide/1 -> Add1/1
  U1/1 -> Divide1/1
  Constant1/1 -> Product/1, Divide/2
  Add/1 -> Divide/1
  [I_uF] -> Add/2
  IU/1 -> Add/1
  Integrator/1 -> U1*/1
  Integrator1/1 -> U2*/1
  Product/1 -> Divide1/2
  Constant4/1 -> Product/2
  Constant3/1 -> Product1/2

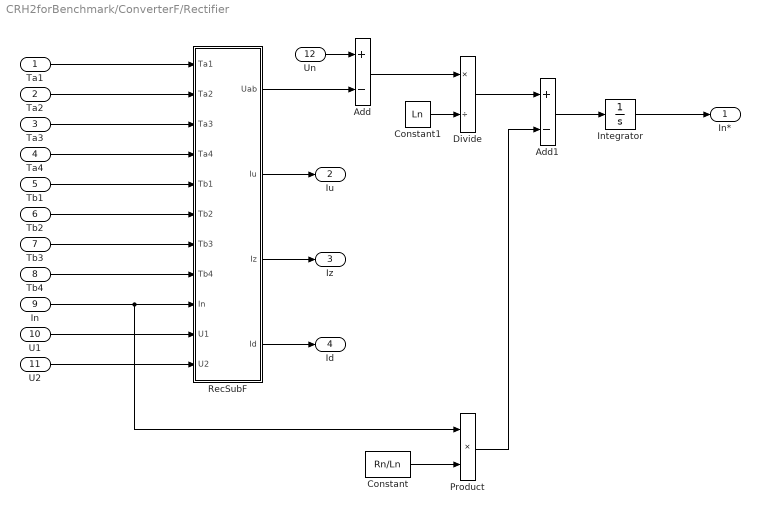
== system CRH2forBenchmark/ConverterF/Rectifier ==
  Ta1 : Inport
  Ta2 : Inport  Port=2
  Ta3 : Inport  Port=3
  Ta4 : Inport  Port=4
  Tb1 : Inport  Port=5
  Tb2 : Inport  Port=6
  Tb3 : Inport  Port=7
  Tb4 : Inport  Port=8
  In : Inport  Port=9
  U1 : Inport  Port=10
  U2 : Inport  Port=11
  Un : Inport  Port=12
  Add : Sum  Inputs=+-  SampleTime=ts
  Add1 : Sum  Inputs=+-  SampleTime=ts
  Constant : Constant  Value=Rn/Ln
  Constant1 : Constant  Value=Ln
  Divide : Product  Inputs=*/  SampleTime=ts
  Integrator : Integrator
  Product : Product  SampleTime=ts
  RecSubF : Subsystem
  In* : Outport
  Iu : Outport  Port=2
  Iz : Outport  Port=3
  Id : Outport  Port=4
  wires:
  RecSubF/4(Id) -> Id/1
  RecSubF/3(Iz) -> Iz/1
  RecSubF/2(Iu) -> Iu/1
  Tb2/1 -> RecSubF/6(Tb2)
  Ta3/1 -> RecSubF/3(Ta3)
  Un/1 -> Add/1
  Tb1/1 -> RecSubF/5(Tb1)
  Tb4/1 -> RecSubF/8(Tb4)
  Tb3/1 -> RecSubF/7(Tb3)
  In/1 -> Product/1, RecSubF/9(In)
  Ta4/1 -> RecSubF/4(Ta4)
  Ta2/1 -> RecSubF/2(Ta2)
  U2/1 -> RecSubF/11(U2)
  Integrator/1 -> In*/1
  Divide/1 -> Add1/1
  U1/1 -> RecSubF/10(U1)
  Constant/1 -> Product/2
  RecSubF/1(Uab) -> Add/2
  Ta1/1 -> RecSubF/1(Ta1)
  Add1/1 -> Integrator/1
  Product/1 -> Add1/2
  Constant1/1 -> Divide/2
  Add/1 -> Divide/1

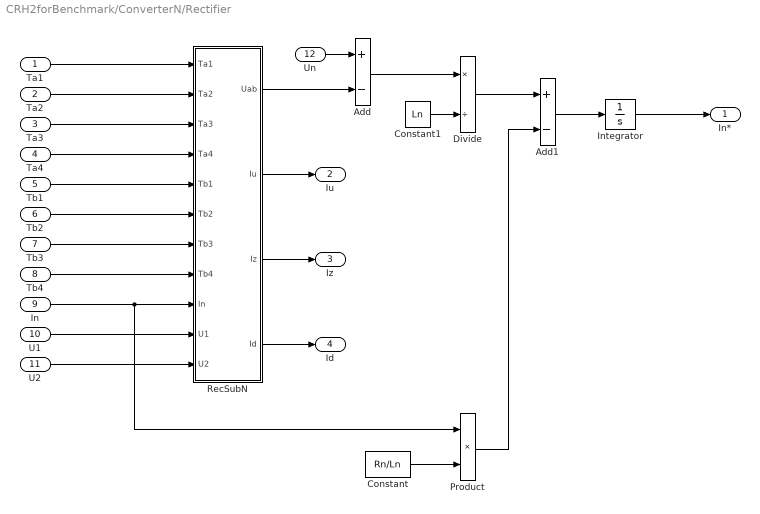
== system CRH2forBenchmark/ConverterN/Rectifier ==
  Ta1 : Inport
  Ta2 : Inport  Port=2
  Ta3 : Inport  Port=3
  Ta4 : Inport  Port=4
  Tb1 : Inport  Port=5
  Tb2 : Inport  Port=6
  Tb3 : Inport  Port=7
  Tb4 : Inport  Port=8
  In : Inport  Port=9
  U1 : Inport  Port=10
  U2 : Inport  Port=11
  Un : Inport  Port=12
  Add : Sum  Inputs=+-  SampleTime=ts
  Add1 : Sum  Inputs=+-  SampleTime=ts
  Constant : Constant  Value=Rn/Ln
  Constant1 : Constant  Value=Ln
  Divide : Product  Inputs=*/  SampleTime=ts
  Integrator : Integrator
  Product : Product  SampleTime=ts
  RecSubN : Subsystem
  In* : Outport
  Iu : Outport  Port=2
  Iz : Outport  Port=3
  Id : Outport  Port=4
  wires:
  Add/1 -> Divide/1
  Constant1/1 -> Divide/2
  Product/1 -> Add1/2
  Add1/1 -> Integrator/1
  Ta1/1 -> RecSubN/1(Ta1)
  RecSubN/1(Uab) -> Add/2
  Constant/1 -> Product/2
  U1/1 -> RecSubN/10(U1)
  Divide/1 -> Add1/1
  Integrator/1 -> In*/1
  U2/1 -> RecSubN/11(U2)
  Ta2/1 -> RecSubN/2(Ta2)
  Ta4/1 -> RecSubN/4(Ta4)
  In/1 -> RecSubN/9(In), Product/1
  Tb3/1 -> RecSubN/7(Tb3)
  Tb4/1 -> RecSubN/8(Tb4)
  Tb1/1 -> RecSubN/5(Tb1)
  Un/1 -> Add/1
  Ta3/1 -> RecSubN/3(Ta3)
  Tb2/1 -> RecSubN/6(Tb2)
  RecSubN/2(Iu) -> Iu/1
  RecSubN/3(Iz) -> Iz/1
  RecSubN/4(Id) -> Id/1

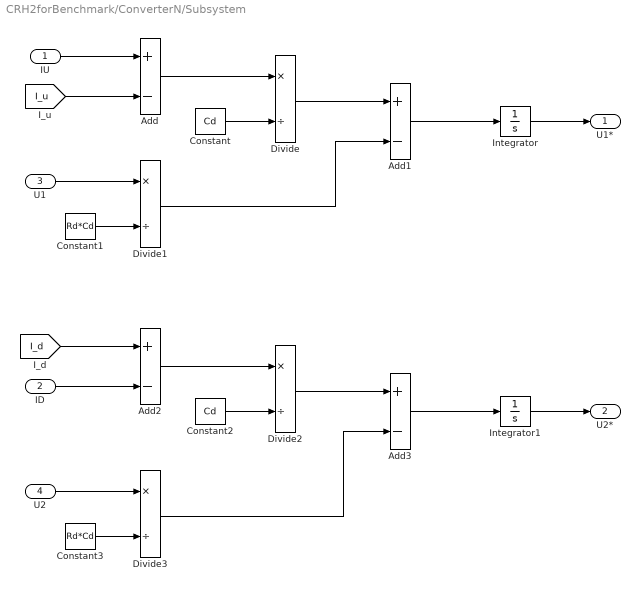
== system CRH2forBenchmark/ConverterN/Subsystem ==
  IU : Inport
  ID : Inport  Port=2
  U1 : Inport  Port=3
  U2 : Inport  Port=4
  Add{,1..3} (4 alike) : Sum  Inputs=+-  SampleTime=ts
  Constant : Constant  Value=Cd
  Constant1 : Constant  Value=Rd*Cd
  Constant2 : Constant  Value=Cd
  Constant3 : Constant  Value=Rd*Cd
  Divide{,1..3} (4 alike) : Product  Inputs=*/
  Integrator : Integrator
  Integrator1 : Integrator
  U1* : Outport
  U2* : Outport  Port=2
  wires:
  Integrator1/1 -> U2*/1
  Integrator/1 -> U1*/1
  IU/1 -> Add/1
  [I_u] -> Add/2
  Add/1 -> Divide/1
  Constant/1 -> Divide/2
  U1/1 -> Divide1/1
  Constant1/1 -> Divide1/2
  Divide/1 -> Add1/1
  Divide1/1 -> Add1/2
  Add1/1 -> Integrator/1
  ID/1 -> Add2/2
  [I_d] -> Add2/1
  Constant2/1 -> Divide2/2
  Add2/1 -> Divide2/1
  Constant3/1 -> Divide3/2
  U2/1 -> Divide3/1
  Divide2/1 -> Add3/1
  Divide3/1 -> Add3/2
  Add3/1 -> Integrator1/1

== system CRH2forBenchmark/DCU1/__InputSSForSFun__ ==
  Commander : Inport
  __UniqueOutportName__1__ : Outport
  __UniqueOutportName__2__ : Outport  Port=2
  __UniqueOutportName__3__ : Outport  Port=3
  __UniqueOutportName__4__ : Outport  Port=4
  __UniqueOutportName__5__ : Outport  Port=5
  __UniqueOutportName__6__ : Outport  Port=6
  __UniqueOutportName__7__ : Outport  Port=7
  __UniqueOutportName__8__ : Outport  Port=8
  __UniqueOutportName__9__ : Outport  Port=9
  wires:
  [w0] -> __UniqueOutportName__9__/1
  [Isabc0] -> __UniqueOutportName__8__/1
  [TL] -> __UniqueOutportName__7__/1
  [Ucd1] -> __UniqueOutportName__6__/1
  [In] -> __UniqueOutportName__5__/1
  [Un] -> __UniqueOutportName__4__/1
  [Ucd2] -> __UniqueOutportName__3__/1
  [Id] -> __UniqueOutportName__2__/1
  Commander/1 -> __UniqueOutportName__1__/1

== system CRH2forBenchmark/DCU1/__OutputSSForSFun__ ==
  __UniqueInportName__1__ : Inport
  __UniqueInportName__2__ : Inport  Port=2
  SPWM1 : Outport
  SPWM : Outport  Port=2
  wires:
  __UniqueInportName__2__/1 -> SPWM/1
  __UniqueInportName__1__/1 -> SPWM1/1

== system CRH2forBenchmark/DCU2/__InputSSForSFun__ ==
  Commander : Inport
  __UniqueOutportName__1__ : Outport
  __UniqueOutportName__2__ : Outport  Port=2
  __UniqueOutportName__3__ : Outport  Port=3
  __UniqueOutportName__4__ : Outport  Port=4
  __UniqueOutportName__5__ : Outport  Port=5
  __UniqueOutportName__6__ : Outport  Port=6
  __UniqueOutportName__7__ : Outport  Port=7
  __UniqueOutportName__8__ : Outport  Port=8
  __UniqueOutportName__9__ : Outport  Port=9
  wires:
  Commander/1 -> __UniqueOutportName__1__/1
  [IdF] -> __UniqueOutportName__2__/1
  [Ucd2F] -> __UniqueOutportName__3__/1
  [UnF] -> __UniqueOutportName__4__/1
  [InF] -> __UniqueOutportName__5__/1
  [Ucd1F] -> __UniqueOutportName__6__/1
  [TLF] -> __UniqueOutportName__7__/1
  [Isabc0F] -> __UniqueOutportName__8__/1
  [w0F] -> __UniqueOutportName__9__/1

== system CRH2forBenchmark/DCU2/__OutputSSForSFun__ ==
  __UniqueInportName__1__ : Inport
  __UniqueInportName__2__ : Inport  Port=2
  SPWM1 : Outport
  SPWM : Outport  Port=2
  wires:
  __UniqueInportName__1__/1 -> SPWM1/1
  __UniqueInportName__2__/1 -> SPWM/1

== system CRH2forBenchmark/IntermediateDClinkF/__InputSSForSFun__ ==
  In1 : Inport
  In2 : Inport  Port=2
  In3 : Inport  Port=3
  In4 : Inport  Port=4
  __UniqueOutportName__1__ : Outport
  __UniqueOutportName__2__ : Outport  Port=2
  __UniqueOutportName__3__ : Outport  Port=3
  __UniqueOutportName__4__ : Outport  Port=4
  wires:
  In1/1 -> __UniqueOutportName__1__/1
  In2/1 -> __UniqueOutportName__2__/1
  In3/1 -> __UniqueOutportName__3__/1
  In4/1 -> __UniqueOutportName__4__/1

== system CRH2forBenchmark/IntermediateDClinkF/__OutputSSForSFun__ ==
  __UniqueInportName__1__ : Inport
  __UniqueInportName__2__ : Inport  Port=2
  __UniqueInportName__3__ : Inport  Port=3
  Out1 : Outport
  Out4 : Outport  Port=2
  Out7 : Outport  Port=3
  wires:
  __UniqueInportName__1__/1 -> Out1/1
  __UniqueInportName__2__/1 -> Out4/1
  __UniqueInportName__3__/1 -> Out7/1

== system CRH2forBenchmark/IntermediateDClinkN/__InputSSForSFun__ ==
  In1 : Inport
  In2 : Inport  Port=2
  In3 : Inport  Port=3
  In4 : Inport  Port=4
  __UniqueOutportName__1__ : Outport
  __UniqueOutportName__2__ : Outport  Port=2
  __UniqueOutportName__3__ : Outport  Port=3
  __UniqueOutportName__4__ : Outport  Port=4
  wires:
  In1/1 -> __UniqueOutportName__1__/1
  In2/1 -> __UniqueOutportName__2__/1
  In3/1 -> __UniqueOutportName__3__/1
  In4/1 -> __UniqueOutportName__4__/1

== system CRH2forBenchmark/IntermediateDClinkN/__OutputSSForSFun__ ==
  __UniqueInportName__1__ : Inport
  __UniqueInportName__2__ : Inport  Port=2
  __UniqueInportName__3__ : Inport  Port=3
  Out1 : Outport
  Out4 : Outport  Port=2
  Out7 : Outport  Port=3
  wires:
  __UniqueInportName__1__/1 -> Out1/1
  __UniqueInportName__2__/1 -> Out4/1
  __UniqueInportName__3__/1 -> Out7/1

== system CRH2forBenchmark/InverterF/InverterTuF ==
  Tu1 : Inport
  Tu2 : Inport  Port=2
  Tu3 : Inport  Port=3
  Tu4 : Inport  Port=4
  Ia : Inport  Port=5
  U1 : Inport  Port=6
  U2 : Inport  Port=7
  InverterTuF_sfcn : S-Function  FunctionName=InverterTuF_sf  SFunctionModules=""  EnableBusSupport=off  mask{rtw_sf_name=InverterTuF_sf, showVar=off}
      mask prompts: rtw_sf_name "Simulink:masks:GenSFuncName_MP"; showVar "Simulink:masks:GenSFuncShowModuleList_MP"
      mask help: Simulink:masks:GenSFuncDesc_MD
      mask init: same as CRH2forBenchmark/DCU1/DCU1_sfcn
      settings: CopyFcn=|
      | if ~strcmp(get_param(gcb,'Linkstatus'),'none') && ...
      | ~strcmp(get_param(gcb,'Linkstatus'),'implicit')
      |   set_param(gcb,'LinkStatus','none');
      | end
      mask Help: eval('feval(''rtwprivate'',''rtwhelpview'',''rtw_sfcn_block'')');
      mask Display:
      | port_label('input',1,'Tu1');
      | port_label('input',2,'Tu2');
      | port_label('input',3,'Tu3');
      | port_label('input',4,'Tu4');
      | port_label('input',5,'Ia');
      | port_label('input',6,'U1');
      | port_label('input',7,'U2');
      | port_label('output',1,'Iu');
      | port_label('output',2,'Iz');
      | port_label('output',3,'Id');
      | port_label('output',4,'Vu');
  __InputSSForSFun__ : Subsystem
  __OutputSSForSFun__ : Subsystem
  Iu : Outport
  Iz : Outport  Port=2
  Id : Outport  Port=3
  Vu : Outport  Port=4
  wires:
  Tu1/1 -> __InputSSForSFun__/1(Tu1)
  Tu2/1 -> __InputSSForSFun__/2(Tu2)
  Tu3/1 -> __InputSSForSFun__/3(Tu3)
  Tu4/1 -> __InputSSForSFun__/4(Tu4)
  Ia/1 -> __InputSSForSFun__/5(Ia)
  U1/1 -> __InputSSForSFun__/6(U1)
  U2/1 -> __InputSSForSFun__/7(U2)
  __InputSSForSFun__/1(__UniqueOutportName__1__) -> InverterTuF_sfcn/1
  __InputSSForSFun__/2(__UniqueOutportName__2__) -> InverterTuF_sfcn/2
  __InputSSForSFun__/3(__UniqueOutportName__3__) -> InverterTuF_sfcn/3
  __InputSSForSFun__/4(__UniqueOutportName__4__) -> InverterTuF_sfcn/4
  __InputSSForSFun__/5(__UniqueOutportName__5__) -> InverterTuF_sfcn/5
  __InputSSForSFun__/6(__UniqueOutportName__6__) -> InverterTuF_sfcn/6
  __InputSSForSFun__/7(__UniqueOutportName__7__) -> InverterTuF_sfcn/7
  InverterTuF_sfcn/1 -> __OutputSSForSFun__/1(__UniqueInportName__1__)
  InverterTuF_sfcn/2 -> __OutputSSForSFun__/2(__UniqueInportName__2__)
  InverterTuF_sfcn/3 -> __OutputSSForSFun__/3(__UniqueInportName__3__)
  InverterTuF_sfcn/4 -> __OutputSSForSFun__/4(__UniqueInportName__4__)
  __OutputSSForSFun__/1(Iu) -> Iu/1
  __OutputSSForSFun__/2(Iz) -> Iz/1
  __OutputSSForSFun__/3(Id) -> Id/1
  __OutputSSForSFun__/4(Vu) -> Vu/1

== system CRH2forBenchmark/InverterF/InverterTvF ==
  Tv1 : Inport
  Tv2 : Inport  Port=2
  Tv3 : Inport  Port=3
  Tv4 : Inport  Port=4
  Ib : Inport  Port=5
  U1 : Inport  Port=6
  U2 : Inport  Port=7
  InverterTvF_sfcn : S-Function  FunctionName=InverterTvF_sf  SFunctionModules=""  EnableBusSupport=off  mask{rtw_sf_name=InverterTvF_sf, showVar=off}
      mask prompts: rtw_sf_name "Simulink:masks:GenSFuncName_MP"; showVar "Simulink:masks:GenSFuncShowModuleList_MP"
      mask help: Simulink:masks:GenSFuncDesc_MD
      mask init: same as CRH2forBenchmark/DCU1/DCU1_sfcn
      settings: CopyFcn=|
      | if ~strcmp(get_param(gcb,'Linkstatus'),'none') && ...
      | ~strcmp(get_param(gcb,'Linkstatus'),'implicit')
      |   set_param(gcb,'LinkStatus','none');
      | end
      mask Help: eval('feval(''rtwprivate'',''rtwhelpview'',''rtw_sfcn_block'')');
      mask Display:
      | port_label('input',1,'Tv1');
      | port_label('input',2,'Tv2');
      | port_label('input',3,'Tv3');
      | port_label('input',4,'Tv4');
      | port_label('input',5,'Ib');
      | port_label('input',6,'U1');
      | port_label('input',7,'U2');
      | port_label('output',1,'Iu');
      | port_label('output',2,'Iz');
      | port_label('output',3,'Id');
      | port_label('output',4,'Vv');
  __InputSSForSFun__ : Subsystem
  __OutputSSForSFun__ : Subsystem
  Iu : Outport
  Iz : Outport  Port=2
  Id : Outport  Port=3
  Vv : Outport  Port=4
  wires:
  Tv1/1 -> __InputSSForSFun__/1(Tv1)
  Tv2/1 -> __InputSSForSFun__/2(Tv2)
  Tv3/1 -> __InputSSForSFun__/3(Tv3)
  Tv4/1 -> __InputSSForSFun__/4(Tv4)
  Ib/1 -> __InputSSForSFun__/5(Ib)
  U1/1 -> __InputSSForSFun__/6(U1)
  U2/1 -> __InputSSForSFun__/7(U2)
  __InputSSForSFun__/1(__UniqueOutportName__1__) -> InverterTvF_sfcn/1
  __InputSSForSFun__/2(__UniqueOutportName__2__) -> InverterTvF_sfcn/2
  __InputSSForSFun__/3(__UniqueOutportName__3__) -> InverterTvF_sfcn/3
  __InputSSForSFun__/4(__UniqueOutportName__4__) -> InverterTvF_sfcn/4
  __InputSSForSFun__/5(__UniqueOutportName__5__) -> InverterTvF_sfcn/5
  __InputSSForSFun__/6(__UniqueOutportName__6__) -> InverterTvF_sfcn/6
  __InputSSForSFun__/7(__UniqueOutportName__7__) -> InverterTvF_sfcn/7
  InverterTvF_sfcn/1 -> __OutputSSForSFun__/1(__UniqueInportName__1__)
  InverterTvF_sfcn/2 -> __OutputSSForSFun__/2(__UniqueInportName__2__)
  InverterTvF_sfcn/3 -> __OutputSSForSFun__/3(__UniqueInportName__3__)
  InverterTvF_sfcn/4 -> __OutputSSForSFun__/4(__UniqueInportName__4__)
  __OutputSSForSFun__/1(Iu) -> Iu/1
  __OutputSSForSFun__/2(Iz) -> Iz/1
  __OutputSSForSFun__/3(Id) -> Id/1
  __OutputSSForSFun__/4(Vv) -> Vv/1

== system CRH2forBenchmark/InverterF/InverterTwF ==
  Tw1 : Inport
  Tw2 : Inport  Port=2
  Tw3 : Inport  Port=3
  Tw4 : Inport  Port=4
  Ic : Inport  Port=5
  U1 : Inport  Port=6
  U2 : Inport  Port=7
  InverterTwF_sfcn : S-Function  FunctionName=InverterTwF_sf  SFunctionModules=""  EnableBusSupport=off  mask{rtw_sf_name=InverterTwF_sf, showVar=off}
      mask prompts: rtw_sf_name "Simulink:masks:GenSFuncName_MP"; showVar "Simulink:masks:GenSFuncShowModuleList_MP"
      mask help: Simulink:masks:GenSFuncDesc_MD
      mask init: same as CRH2forBenchmark/DCU1/DCU1_sfcn
      settings: CopyFcn=|
      | if ~strcmp(get_param(gcb,'Linkstatus'),'none') && ...
      | ~strcmp(get_param(gcb,'Linkstatus'),'implicit')
      |   set_param(gcb,'LinkStatus','none');
      | end
      mask Help: eval('feval(''rtwprivate'',''rtwhelpview'',''rtw_sfcn_block'')');
      mask Display:
      | port_label('input',1,'Tw1');
      | port_label('input',2,'Tw2');
      | port_label('input',3,'Tw3');
      | port_label('input',4,'Tw4');
      | port_label('input',5,'Ic');
      | port_label('input',6,'U1');
      | port_label('input',7,'U2');
      | port_label('output',1,'Iu');
      | port_label('output',2,'Iz');
      | port_label('output',3,'Id');
      | port_label('output',4,'Vw');
  __InputSSForSFun__ : Subsystem
  __OutputSSForSFun__ : Subsystem
  Iu : Outport
  Iz : Outport  Port=2
  Id : Outport  Port=3
  Vw : Outport  Port=4
  wires:
  Tw1/1 -> __InputSSForSFun__/1(Tw1)
  Tw2/1 -> __InputSSForSFun__/2(Tw2)
  Tw3/1 -> __InputSSForSFun__/3(Tw3)
  Tw4/1 -> __InputSSForSFun__/4(Tw4)
  Ic/1 -> __InputSSForSFun__/5(Ic)
  U1/1 -> __InputSSForSFun__/6(U1)
  U2/1 -> __InputSSForSFun__/7(U2)
  __InputSSForSFun__/1(__UniqueOutportName__1__) -> InverterTwF_sfcn/1
  __InputSSForSFun__/2(__UniqueOutportName__2__) -> InverterTwF_sfcn/2
  __InputSSForSFun__/3(__UniqueOutportName__3__) -> InverterTwF_sfcn/3
  __InputSSForSFun__/4(__UniqueOutportName__4__) -> InverterTwF_sfcn/4
  __InputSSForSFun__/5(__UniqueOutportName__5__) -> InverterTwF_sfcn/5
  __InputSSForSFun__/6(__UniqueOutportName__6__) -> InverterTwF_sfcn/6
  __InputSSForSFun__/7(__UniqueOutportName__7__) -> InverterTwF_sfcn/7
  InverterTwF_sfcn/1 -> __OutputSSForSFun__/1(__UniqueInportName__1__)
  InverterTwF_sfcn/2 -> __OutputSSForSFun__/2(__UniqueInportName__2__)
  InverterTwF_sfcn/3 -> __OutputSSForSFun__/3(__UniqueInportName__3__)
  InverterTwF_sfcn/4 -> __OutputSSForSFun__/4(__UniqueInportName__4__)
  __OutputSSForSFun__/1(Iu) -> Iu/1
  __OutputSSForSFun__/2(Iz) -> Iz/1
  __OutputSSForSFun__/3(Id) -> Id/1
  __OutputSSForSFun__/4(Vw) -> Vw/1

== system CRH2forBenchmark/InverterF/Pulse ==
  note: PhaseA:1 to 4
      |
      | PhaseB:5 to 8
      |
      | PhaseC:9 to 12
  State : Inport
  Add : Sum
  Constant : Constant  Value=2
  Demux : Demux  Outputs=3
  Multiport Switch : MultiPortSwitch
  Multiport Switch1 : MultiPortSwitch
  Multiport Switch2 : MultiPortSwitch
  Mux : Mux  Inputs=3
  S =  Ud : Constant  Value=[1 1 0 0]
  S = - Ud : Constant  Value=[0 0 1 1]
  S = 0 : Constant  Value=[0 1 1 0]
  SVPWM : Outport
  wires:
  Add/1 -> Demux/1
  Multiport Switch1/1 -> Mux/2
  S = 0/1 -> Multiport Switch/3, Multiport Switch1/3, Multiport Switch2/3
  Demux/2 -> Multiport Switch1/1
  Demux/3 -> Multiport Switch2/1
  State/1 -> Add/1
  Constant/1 -> Add/2
  Mux/1 -> SVPWM/1
  Demux/1 -> Multiport Switch/1
  Multiport Switch2/1 -> Mux/3
  S =  Ud/1 -> Multiport Switch/4, Multiport Switch1/4, Multiport Switch2/4
  Multiport Switch/1 -> Mux/1
  S = - Ud/1 -> Multiport Switch1/2, Multiport Switch/2, Multiport Switch2/2
